simulink model "control_diagram_previous"  (R2018a)
settings: Solver=VariableStepAuto  StartTime=0.0  StopTime=50.0  RelTol=1e-3
values from neighbouring files (symbols this model uses):
  w1 = vector_bases(9)    [custo_fli.m]    (also in custo_total.m; planta_final.m)
  w2 = vector_bases(10)    [custo_fli.m]    (also in custo_total.m; planta_final.m)
libraries: fuzblock x3
settings Model: Creator=root  LastModifiedBy=User
settings DebuggingCC: LibraryContextMissingDiagnostic=warning
settings SFSimCC: SimUseLocalCustomCode=on
settings RTWCC: RTWUseLocalCustomCode=on

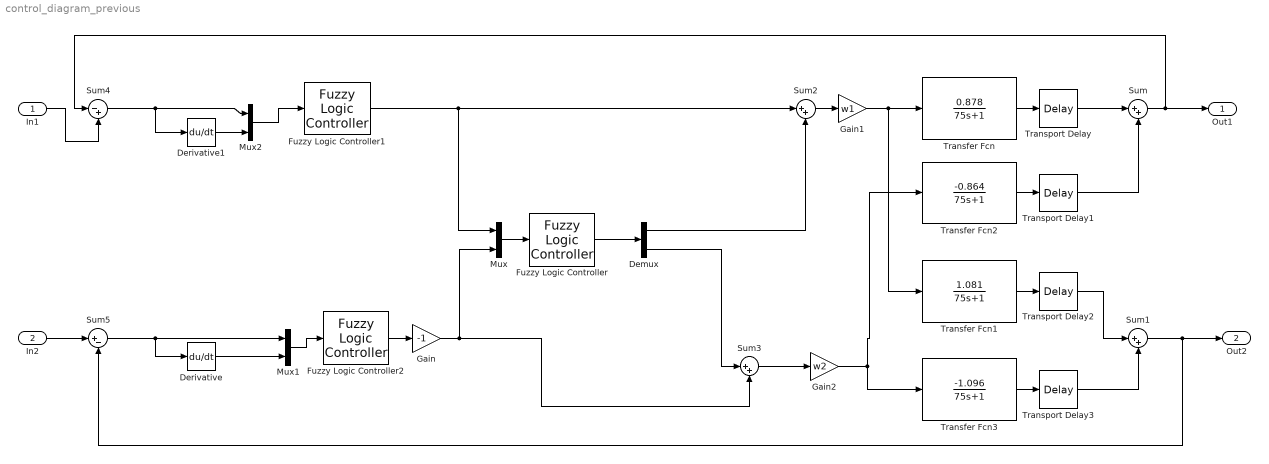
== system control_diagram_previous ==
  In1 : Inport
  In2 : Inport  Port=2
  Demux : Demux  Outputs=2
  Derivative : Derivative
  Derivative1 : Derivative
  Fuzzy Logic Controller : fuzblock/Fuzzy Logic  Controller  FIS='tipper.fis'  OutputSampleNumber=101  DataType=double  FuzzifiedInputs=off  RuleFiringStrengths=off  RuleOutputs=off  AggregatedOutputs=off  SimulateUsing=Interpreted execution  OutOfRangeInputValueMessage=warning  NoRuleFiredMessage=warning  EmptyOutputFuzzySetMessage=warning
  Fuzzy Logic Controller1 : fuzblock/Fuzzy Logic  Controller  FIS=flc1  OutputSampleNumber=101  DataType=double  FuzzifiedInputs=off  RuleFiringStrengths=off  RuleOutputs=off  AggregatedOutputs=off  SimulateUsing=Interpreted execution  OutOfRangeInputValueMessage=warning  NoRuleFiredMessage=warning  EmptyOutputFuzzySetMessage=warning
  Fuzzy Logic Controller2 : fuzblock/Fuzzy Logic  Controller  FIS=flc2  OutputSampleNumber=101  DataType=double  FuzzifiedInputs=off  RuleFiringStrengths=off  RuleOutputs=off  AggregatedOutputs=off  SimulateUsing=Interpreted execution  OutOfRangeInputValueMessage=warning  NoRuleFiredMessage=warning  EmptyOutputFuzzySetMessage=warning
  Gain : Gain  Gain=-1
  Gain1 : Gain  Gain=w1
  Gain2 : Gain  Gain=w2
  Mux : Mux  Inputs=2
  Mux1 : Mux  Inputs=2
  Mux2 : Mux  Inputs=2
  Sum{,1..3} (4 alike) : Sum  Inputs=|++
  Sum4 : Sum  Inputs=|-+
  Sum5 : Sum  Inputs=|+-
  Transfer Fcn : TransferFcn  Numerator=[0.878]  Denominator=[75 1]
  Transfer Fcn1 : TransferFcn  Numerator=[1.081]  Denominator=[75 1]
  Transfer Fcn2 : TransferFcn  Numerator=[-0.864]  Denominator=[75 1]
  Transfer Fcn3 : TransferFcn  Numerator=[-1.096]  Denominator=[75 1]
  Transport Delay{,1..3} (4 alike) : TransportDelay
  Out1 : Outport  SignalName=y1
  Out2 : Outport  Port=2  SignalName=y2
  wires:
  Transfer Fcn/1 -> Transport Delay/1
  Transfer Fcn2/1 -> Transport Delay1/1
  Transport Delay1/1 -> Sum/2
  Transport Delay/1 -> Sum/1
  Sum/1 -> Sum4/1, Out1/1
  Transfer Fcn1/1 -> Transport Delay2/1
  Transfer Fcn3/1 -> Transport Delay3/1
  Transport Delay2/1 -> Sum1/1
  Transport Delay3/1 -> Sum1/2
  Fuzzy Logic Controller/1 -> Demux/1
  Mux/1 -> Fuzzy Logic Controller/1
  Fuzzy Logic Controller1/1 -> Sum2/1, Mux/1
  Demux/1 -> Sum2/2
  Demux/2 -> Sum3/1
  Fuzzy Logic Controller2/1 -> Gain/1
  Sum3/1 -> Gain2/1
  Sum2/1 -> Gain1/1
  Sum1/1 -> Sum5/2, Out2/1
  In1/1 -> Sum4/2
  In2/1 -> Sum5/1
  Sum5/1 -> Derivative/1, Mux1/1
  Derivative/1 -> Mux1/2
  Mux1/1 -> Fuzzy Logic Controller2/1
  Mux2/1 -> Fuzzy Logic Controller1/1
  Derivative1/1 -> Mux2/2
  Sum4/1 -> Derivative1/1, Mux2/1
  Gain/1 -> Sum3/2, Mux/2
  Gain1/1 -> Transfer Fcn1/1, Transfer Fcn/1
  Gain2/1 -> Transfer Fcn2/1, Transfer Fcn3/1
